simulink model "heatex_sim"  (Simulink 4.00)
settings: Solver=ode4  StartTime=0.0  StopTime=200  FixedStep=2  RelTol=1e-3
StartFcn:
  | heatex_clbk('Start')
StopFcn:
  | heatex_clbk('Stop')
libraries: cstblocks x4, simulink3 x2
CloseFcn:
  | heatex_clbk('Close')
settings Model: LastModifiedBy=nhickey  SaveTime=off  SaveOutput=off  BlockReductionOpt=off

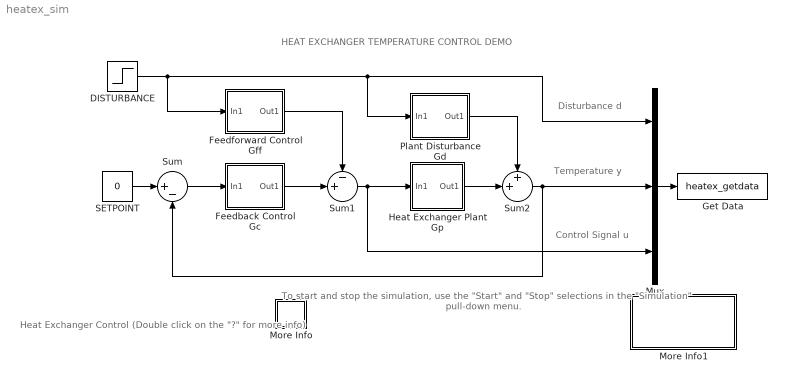
== system heatex_sim ==
  note: HEAT EXCHANGER TEMPERATURE CONTROL DEMO
  note: Control Signal u
  note: Temperature y
  note: Disturbance d
  note: Heat Exchanger Control
      | (Double click on the "?" for more info)
  note: To start and stop the simulation, use the "Start" and
      | "Stop" selections in the "Simulation" pull-down menu.
  DISTURBANCE : Step  Time=20  Before=0  After=-1  SampleTime=0
  Feedback Control Gc : Subsystem
      settings: RTWFcnNameOpts=Auto  RTWFileNameOpts=Auto
  Feedforward Control Gff : Subsystem
      settings: RTWFcnNameOpts=Auto  RTWFileNameOpts=Auto
  Get Data : S-Function  FunctionName=heatex_getdata  PortCounts=[]  SFunctionModules=''
  Heat Exchanger Plant Gp : Subsystem
      settings: RTWFcnNameOpts=Auto  RTWFileNameOpts=Auto
  More Info : Subsystem
      settings: RTWFcnNameOpts=Auto  RTWFileNameOpts=Auto
      mask Display: disp('?')
  More Info1 : Subsystem
      settings: OpenFcn=simcad(bdroot);  RTWFcnNameOpts=Auto  RTWFileNameOpts=Auto
      mask Display: disp('Double click\nhere for\nSimulink Help')
  Mux : Mux  Inputs=3
  Plant Disturbance Gd : Subsystem
      settings: RTWFcnNameOpts=Auto  RTWFileNameOpts=Auto
  SETPOINT : Constant  Value=0
  Sum : Sum  Inputs=|+-  SaturateOnIntegerOverflow=on
  Sum1 : Sum  Inputs=-+|  SaturateOnIntegerOverflow=on
  Sum2 : Sum  Inputs=++|  SaturateOnIntegerOverflow=on
  wires:
  SETPOINT/1 -> Sum/1
  Sum/1 -> Feedback Control Gc/1(In1)
  Sum1/1 -> Heat Exchanger Plant Gp/1(In1), Mux/3
  Sum2/1 -> Sum/2, Mux/2
  Mux/1 -> Get Data/1
  Feedforward Control Gff/1(Out1) -> Sum1/1
  DISTURBANCE/1 -> Feedforward Control Gff/1(In1), Mux/1, Plant Disturbance Gd/1(In1)
  Feedback Control Gc/1(Out1) -> Sum1/2
  Heat Exchanger Plant Gp/1(Out1) -> Sum2/2
  Plant Disturbance Gd/1(Out1) -> Sum2/1

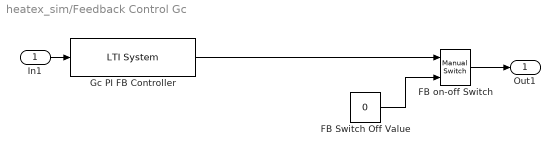
== system heatex_sim/Feedback Control Gc ==
  In1 : Inport  Port=1
  FB Switch Off Value : Constant  Value=0
  FB on-off Switch : simulink3/Nonlinear/Manual Switch  sw=1  action=0
  Gc PI FB Controller : cstblocks/LTI System  sys=tf([30.31 1.23],[24.56 0])  IC=0
  Out1 : Outport  Port=1
  wires:
  In1/1 -> Gc PI FB Controller/1
  Gc PI FB Controller/1 -> FB on-off Switch/1
  FB on-off Switch/1 -> Out1/1
  FB Switch Off Value/1 -> FB on-off Switch/2

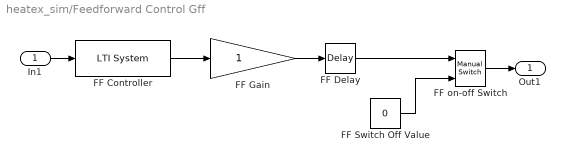
== system heatex_sim/Feedforward Control Gff ==
  In1 : Inport  Port=1
  FF Controller : cstblocks/LTI System  sys=tf([21.3 1],[25 1])  IC=0
  FF Delay : TransportDelay  DelayTime=25.3  InitialInput=0  BufferSize=1024  PadeOrder=0
      settings: CloseFcn=disp('hello')
  FF Gain : Gain  Gain=1  Multiplication=Element-wise(K.*u)  SaturateOnIntegerOverflow=on
      settings: CloseFcn=disp('hello')
  FF Switch Off Value : Constant  Value=0
  FF on-off Switch : simulink3/Nonlinear/Manual Switch  sw=0  action=0
  Out1 : Outport  Port=1
  wires:
  In1/1 -> FF Controller/1
  FF Gain/1 -> FF Delay/1
  FF Controller/1 -> FF Gain/1
  FF Delay/1 -> FF on-off Switch/1
  FF on-off Switch/1 -> Out1/1
  FF Switch Off Value/1 -> FF on-off Switch/2

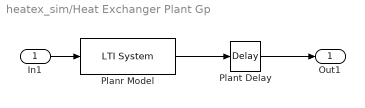
== system heatex_sim/Heat Exchanger Plant Gp ==
  In1 : Inport  Port=1
  Planr Model : cstblocks/LTI System  sys=tf(1,[21.3 1])  IC=0
  Plant Delay : TransportDelay  DelayTime=14.7  InitialInput=0  BufferSize=1024  PadeOrder=0
  Out1 : Outport  Port=1
  wires:
  In1/1 -> Planr Model/1
  Planr Model/1 -> Plant Delay/1
  Plant Delay/1 -> Out1/1

== system heatex_sim/More Info ==
  note: Try experimenting with switching between
      | using Feedforward and/or Feedback control.
      | Type heatex at the MATLAB prompt to see the demo.
  note: This demonstration shows the temperature control of a continuous stirred
      | tank reactor (CSTR) using a heat exchanger.
      | The controllers have been designed to regulate the temperature of the
      | liquid in the tank when subject to disturbances in the temperature of inlet flow.

== system heatex_sim/More Info1 ==

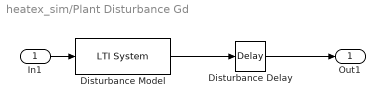
== system heatex_sim/Plant Disturbance Gd ==
  In1 : Inport  Port=1
  Disturbance Delay : TransportDelay  DelayTime=35  InitialInput=0  BufferSize=1024  PadeOrder=0
  Disturbance Model : cstblocks/LTI System  sys=tf(1,[25 1])  IC=0
  Out1 : Outport  Port=1
  wires:
  Disturbance Delay/1 -> Out1/1
  In1/1 -> Disturbance Model/1
  Disturbance Model/1 -> Disturbance Delay/1
